simulink model "CTRL_TRGT_YRDES_test"  (R2023b)
settings: Solver=VariableStepAuto  StartTime=0.0  StopTime=10.0  RelTol=1e-3
libraries: CTRL_TRGT_YRDES x1
settings Model: Creator=blatak  LastModifiedBy=blatak

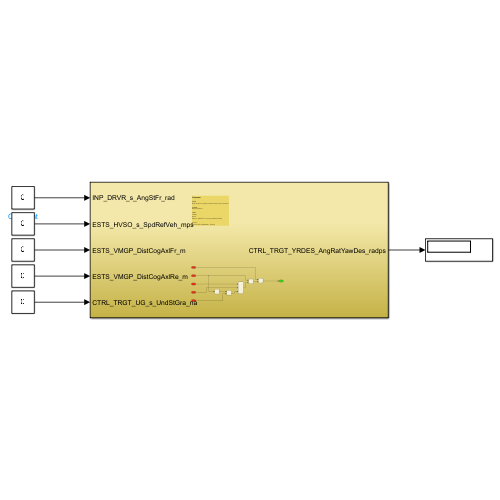
[thumbnail: Simulink's stored preview of the top-level diagram]
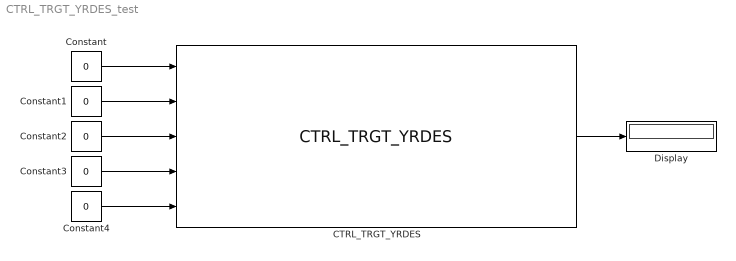
== system CTRL_TRGT_YRDES_test ==
  CTRL_TRGT_YRDES : CTRL_TRGT_YRDES/CTRL_TRGT_YRDES  SystemSampleTime=-1  VariantActivationTime=update diagram  AllowFlexibleInterface=on  Latency=0  AutoFrameSizeCalculation=off
  Constant{,1..4} (5 alike) : Constant  Value=0  OutDataTypeStr=single
  Display : Display
  wires:
  Constant/1 -> CTRL_TRGT_YRDES/1
  Constant1/1 -> CTRL_TRGT_YRDES/2
  Constant2/1 -> CTRL_TRGT_YRDES/3
  Constant3/1 -> CTRL_TRGT_YRDES/4
  Constant4/1 -> CTRL_TRGT_YRDES/5
  CTRL_TRGT_YRDES/1 -> Display/1
